simulink model "Pendulum24_state_prefilter"  (R2024a)
settings: Solver=ode45  StartTime=0.0  StopTime=20  MaxStep=1e-2  RelTol=1e-3  EnableMultiTasking=on
InitFcn:
  | g = 9.81; %gravitational constant
  | 
  | %% S-function
  | % showVR = 0;
  | % CartBlocking = 0;
  | % CartHard = 0;
  | % phi0 = 0; %initial conditions
values from neighbouring files (symbols this model uses):
  A_down = double(subs(A_sym, [X; u], [X_down; u_eq]))    [linearization.m]    (also in my_pendulum.m)
  A_up = double(subs(A_sym, [X; u], [X_up; u_eq]))    [linearization.m]    (also in my_pendulum.m)
  B_down = double(subs(B_sym, [X; u], [X_down; u_eq]))    [linearization.m]    (also in my_pendulum.m)
  B_up = double(subs(B_sym, [X; u], [X_up; u_eq]))    [linearization.m]    (also in my_pendulum.m)
  C_four = eye(4)    [linearization.m]    (also in my_pendulum.m)
  D_four = zeros(4, 1)    [linearization.m]    (also in my_pendulum.m)
  K_down = place(A_down, B_down, p_des)    [linearization.m]    (also in my_pendulum.m = place(A_down, B_down, p_down))
  K_up = lqr(A_up, B_up, Q, R)    [linearization.m]    (also in my_pendulum.m = place(A_up, B_up, p_up))
  M_down = -1 / (C_y * inv(A_down - B_down * K_down) * B_down)    [linearization.m]    (also in my_pendulum.m)
  M_up = -1 / (C_y_up * inv(A_up - B_up * K_up) * B_up)    [linearization.m]    (also in my_pendulum.m = -1 / (C_y * inv(A_up - B_up * K_up) * B_up))
libraries: vrlib x4
CloseFcn:
  | vrclose all;
  | clear figureVR worldVR;
settings Model: Creator=H  LastModifiedBy=jx2004
settings SolverCC: AlgebraicLoopSolver=TrustRegion
settings DataIOCC: LimitDataPoints=on  SaveFormat=Array  SignalLoggingSaveFormat=ModelDataLogs  ReturnWorkspaceOutputs=off
settings OptimizationCC: ExpressionDepthLimit=2147483647  InitFltsAndDblsToZero=on  LifeSpan=inf
settings DebuggingCC: SaveWithParameterizedLinksMsg=none  UnderspecifiedInitializationDetection=Classic  MergeDetectMultiDrivingBlocksExec=none  SignalResolutionControl=TryResolveAllWithWarning  SolverPrmCheckMsg=warning  FcnCallInpInsideContextMsg=warning  UnconnectedInputMsg=warning  UnconnectedOutputMsg=warning  UnconnectedLineMsg=warning  StateNameClashWarn=warning  SFUnexpectedBacktrackingDiag=warning  SFNoUnconditionalDefaultTransitionDiag=warning  SFExecutionAtInitializationDiag=none  ArithmeticOperatorsInVariantConditions=warning
settings HardwareCC: ProdBitPerPointer=32  ProdBitPerSizeT=32  ProdBitPerPtrDiffT=32  ProdLargestAtomicFloat=None  ProdIntDivRoundTo=Undefined  ProdEndianess=Unspecified  ProdWordSize=32  ProdHWDeviceType=32-bit Generic
settings ModelReferenceCC: PropagateSignalLabelsOutOfModel=off
settings SFSimCC: SimUseLocalCustomCode=off  CustomCodeUndefinedFunction=UseInterfaceOnly
settings RTWCC: RTWUseLocalCustomCode=off  GPUComputeCapability=3.5
settings CodeAppCC: StateflowObjectComments=on
settings GRTTargetCC: TargetFcnLib=ansi_tfl_tmw.mat  TargetLangStandard=C89/C90 (ANSI)  CombineOutputUpdateFcns=off  GRTInterface=on
settings ConfigComp: CovMetricSettings=dw  CovSaveCumulativeToWorkspaceVar=on  CovSaveSingleToWorkspaceVar=on  CovExternalEMLEnable=off

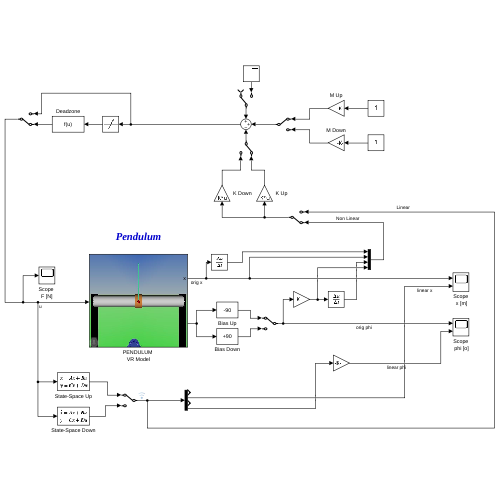
[thumbnail: Simulink's stored preview of the top-level diagram]
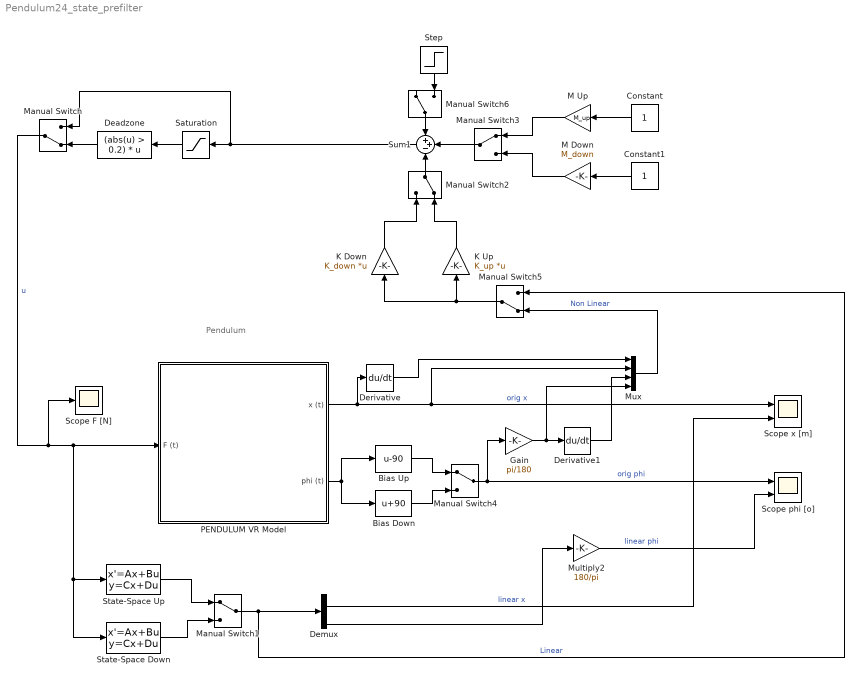
== system Pendulum24_state_prefilter ==
  note: Pendulum
  Bias Down : Bias  Bias=90  SaturateOnIntegerOverflow=off
  Bias Up : Bias  Bias=-90  SaturateOnIntegerOverflow=off
  Constant : Constant
  Constant1 : Constant
  Deadzone : Fcn  Expr=(abs(u) > 0.2) * u
  Demux : Demux
  Derivative : Derivative
  Derivative1 : Derivative
  Gain : Gain  Gain=pi/180
  K Down : Gain  Gain=K_down  Multiplication=Matrix(K*u)
  K Up : Gain  Gain=K_up  Multiplication=Matrix(K*u)
  M Down : Gain  Gain=M_down
  M Up : Gain  Gain=M_up
  Manual Switch : ManualSwitch  CurrentSetting=0
  Manual Switch{1,3..4,6} (4 alike) : ManualSwitch
  Manual Switch2 : ManualSwitch  CurrentSetting=0
  Manual Switch5 : ManualSwitch  CurrentSetting=0
  Multiply2 : Gain  Gain=180/pi
  Mux : Mux
  PENDULUM VR Model : Subsystem  mask(Pendulum){showVR=on, phi0=90, y0=0, brake=off, rail_bound=off}
      mask prompts: showVR "Show Virtual World?"; phi0 "Initial angle of the pendulum   phi(0) [deg] (from horizontal plane)"; y0 "Initial position of the cart x0 [m] (rightwise from the center)"; brake "Cart brake"; rail_bound "Obey rail boundaries"
      mask help: Pendulum - Virtual Reality
      mask init:
      | clear figureVR worldVR;
      | showVR = 1;
      mask Help:
      | Pendulum - Virtual Reality. <br><br>
      | 
      | This is a model of the inverted pendulum on a cart, which consit of a beam and a cart. The beam is connected with the cart by a pivot. The input of this system is mechanical force applied on the cart, outputs are the angle of the beam and the position of the cart.   <br><br>
      | 
      | 
      | In the mask of the model, it can be set:
      | <ul>
      | <li>Initial angle of the pendulum</li>
      | </ul><br><br>
      | 
      | 
      | Copyright: 2007,   Jan Vana, Jirka Roubal, Petr Husek.
      mask Callback showVR:
      | if strcmp('off',get_param(gcb,'showVR'))
      |     vrclose all;
      | else
      |     if exist('figureVR')==0
      |         figureVR = vrfigure;
      |     end
      |     if exist('worldVR')==0
      |         worldVR = vrworld('Pendulum_VR.WRL');
      |     end
      | 	if isvalid(figureVR)==0
      |         open(worldVR);
      |         figureVR = vrfigure(worldVR,[650 80 550 350]);
      | 	end
      | end
      mask Display:
      | image(imread('Pendulum_Image.jpg'))
      | port_label ('input',1,'F')
      | port_label ('output',1,'x')
      | port_label ('output',2,'phi')
  Saturation : Saturate  UpperLimit=10  LowerLimit=-10
  Scope phi [o] : Scope  NumInputPorts=2
  Scope x [m] : Scope  NumInputPorts=2
  Scope F [N] : Scope
  State-Space Down : StateSpace  A=A_down  B=B_down  C=C_four  D=D_four  InitialCondition=[0; 0; 0; 0]
  State-Space Up : StateSpace  A=A_up  B=B_up  C=C_four  D=D_four  InitialCondition=[0; 0; 0; 0]
  Step : Step  SampleTime=2
  Sum1 : Sum  Inputs=++-
  wires:
  Manual Switch/1 -> Scope F [N]/1, State-Space Down/1, State-Space Up/1, PENDULUM VR Model/1(F (t))  "u"
  PENDULUM VR Model/2(phi (t)) -> Bias Up/1, Bias Down/1
  Multiply2/1 -> Scope phi [o]/2  "linear phi"
  PENDULUM VR Model/1(x (t)) -> Derivative/1, Scope x [m]/1, Mux/2  "orig x"
  Deadzone/1 -> Manual Switch/2
  Saturation/1 -> Deadzone/1
  Sum1/1 -> Manual Switch/1, Saturation/1
  Demux/4 -> Multiply2/1
  Demux/2 -> Scope x [m]/2  "linear x"
  Manual Switch1/1 -> Manual Switch5/1, Demux/1  "Linear"
  State-Space Up/1 -> Manual Switch1/1
  State-Space Down/1 -> Manual Switch1/2
  K Down/1 -> Manual Switch2/1
  K Up/1 -> Manual Switch2/2
  M Down/1 -> Manual Switch3/2
  M Up/1 -> Manual Switch3/1
  Constant/1 -> M Up/1
  Constant1/1 -> M Down/1
  Manual Switch3/1 -> Sum1/2
  Manual Switch2/1 -> Sum1/3
  Manual Switch4/1 -> Gain/1, Scope phi [o]/1  "orig phi"
  Bias Up/1 -> Manual Switch4/1
  Bias Down/1 -> Manual Switch4/2
  Derivative/1 -> Mux/1
  Manual Switch5/1 -> K Down/1, K Up/1
  Mux/1 -> Manual Switch5/2  "Non Linear"
  Gain/1 -> Mux/4, Derivative1/1
  Derivative1/1 -> Mux/3
  Manual Switch6/1 -> Sum1/1
  Step/1 -> Manual Switch6/2

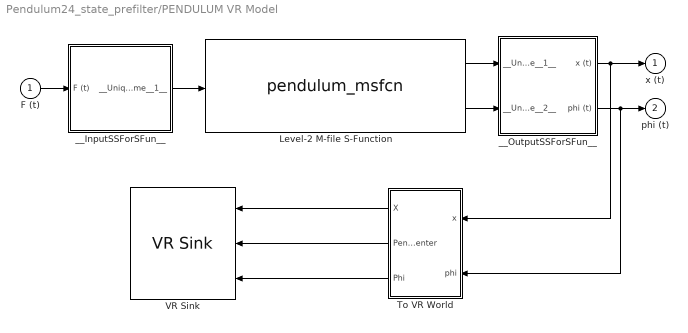
== system Pendulum24_state_prefilter/PENDULUM VR Model ==
  F (t) : Inport
  Level-2 M-file S-Function : M-S-Function  FunctionName=pendulum_msfcn  Parameters=y0, phi0, rail_bound, brake
  To VR World : Subsystem
  VR Sink : vrlib/VR Sink  InstantiateOnLoad=on  SampleTime=0.1  ViewEnable=on  RemoteChange=off  RemoteView=on  FieldsWritten=cart.translation.3.1.double#pendulum.center.3.1.double#pendulum.rotation.4.1.double  WorldFileName=Pendulum_VR.WRL  AutoView=off  VideoDimensions=[]  AllowVariableSize=off
  __InputSSForSFun__ : Subsystem
  __OutputSSForSFun__ : Subsystem
  x (t) : Outport  OutDataTypeStr=double  PortDimensions=1  SampleTime=[-1 0]
  phi (t) : Outport  Port=2  OutDataTypeStr=double  PortDimensions=1  SampleTime=[-1 0]
  wires:
  To VR World/1(X) -> VR Sink/1
  To VR World/2(Pend center) -> VR Sink/2
  To VR World/3(Phi) -> VR Sink/3
  __OutputSSForSFun__/2(phi (t)) -> To VR World/2(phi), phi (t)/1
  __OutputSSForSFun__/1(x (t)) -> To VR World/1(x), x (t)/1
  Level-2 M-file S-Function/2 -> __OutputSSForSFun__/2(__UniqueInportName__2__)
  Level-2 M-file S-Function/1 -> __OutputSSForSFun__/1(__UniqueInportName__1__)
  __InputSSForSFun__/1(__UniqueOutportName__1__) -> Level-2 M-file S-Function/1
  F (t)/1 -> __InputSSForSFun__/1(F (t))

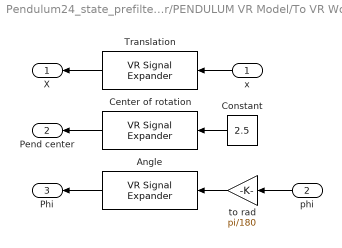
== system Pendulum24_state_prefilter/PENDULUM VR Model/To VR World ==
  x : Inport
  phi : Inport  Port=2
  Angle : vrlib/VR Signal Expander  outwidth=4  outidx=[4]
  Center of rotation : vrlib/VR Signal Expander  outwidth=3  outidx=[2]
  Constant : Constant  Value=2.5
  Translation : vrlib/VR Signal Expander  outwidth=3  outidx=[1]
  to rad : Gain  Gain=pi/180
  X : Outport
  Pend center : Outport  Port=2
  Phi : Outport  Port=3
  wires:
  Angle/1 -> Phi/1
  Center of rotation/1 -> Pend center/1
  Translation/1 -> X/1
  phi/1 -> to rad/1
  x/1 -> Translation/1
  to rad/1 -> Angle/1
  Constant/1 -> Center of rotation/1

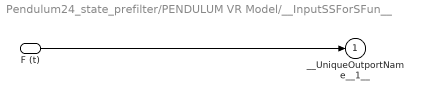
== system Pendulum24_state_prefilter/PENDULUM VR Model/__InputSSForSFun__ ==
  F (t) : Inport
  __UniqueOutportName__1__ : Outport
  wires:
  F (t)/1 -> __UniqueOutportName__1__/1

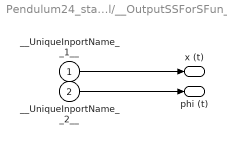
== system Pendulum24_state_prefilter/PENDULUM VR Model/__OutputSSForSFun__ ==
  __UniqueInportName__1__ : Inport
  __UniqueInportName__2__ : Inport  Port=2
  x (t) : Outport  OutDataTypeStr=double  PortDimensions=1  SampleTime=[-1 0]
  phi (t) : Outport  Port=2  OutDataTypeStr=double  PortDimensions=1  SampleTime=[-1 0]
  wires:
  __UniqueInportName__2__/1 -> phi (t)/1
  __UniqueInportName__1__/1 -> x (t)/1
